simulink model "sampleModel1508"  (R2023a)
settings: Solver=VariableStepAuto  StartTime=0.0  StopTime=10.0  RelTol=1e-3
libraries: hdlsllib x4, simulink x3
settings Model: Creator=user1  LastModifiedBy=user1

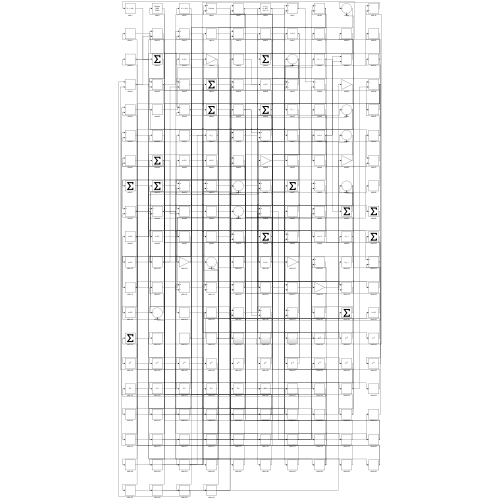
[thumbnail: Simulink's stored preview of the top-level diagram]
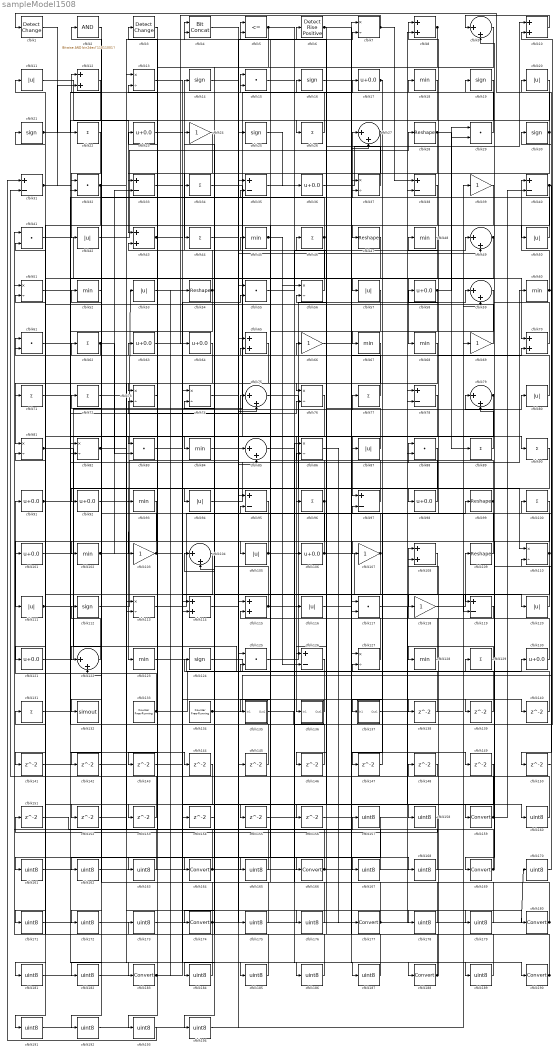
== system sampleModel1508 ==
  cfblk1 : simulink/Logic and Bit Operations/Detect Change  vinit=0  OutDataTypeStr=boolean
      settings: LibrarySourceBlock=|
      | hdlsllib/Logic and Bit
      | Operations/Detect
      | Change
  cfblk{8,10,12,43,65,70,108,114..115} (9 alike) : Sum
  cfblk{22,26,34,44,46,62,71..72,77,89..90,96,100,129,131} (15 alike) : Sum  Inputs=+
  cfblk{17,23,36,58,63..64,91..92,98,101,106,121,130} (13 alike) : Bias  Bias=0.0  SaturateOnIntegerOverflow=off
  cfblk{18,45,48,52,60,67..68,84,93,102,123,128} (12 alike) : MinMax
  cfblk{24,39,66,69,103,107,118} (7 alike) : Gain
  cfblk{9,27,49,59,75,79,85,104,122} (9 alike) : Sum  Inputs=|++
  cfblk{11,20,42,50,53,57,80,87,94,105,111,116,120} (13 alike) : Abs  SaturateOnIntegerOverflow=off
  cfblk{28,47,54,99,109} (5 alike) : Reshape
  cfblk{7,13,37,51,56,73..74,76,81..82,86,110,113,127} (14 alike) : Product  Inputs=*/  RndMeth=Zero  SaturateOnIntegerOverflow=on
  cfblk{14,16,19,21,25,30,112,124} (8 alike) : Signum
  cfblk{15,29,32,41,55,61,83,88,117,125} (10 alike) : DotProduct  OutDataTypeStr=Inherit: Inherit via internal rule
  cfblk{31,33,35,38,40,78,95,97,119,126} (10 alike) : Sum  Inputs=+-
  cfblk132 : ToWorkspace  VariableName=simout  SaveFormat=Timeseries  SampleTime=-1
  cfblk133 : hdlsllib/Sources/Counter Free-Running  NumBits=16  tsamp=-1
  cfblk134 : hdlsllib/Sources/Counter Free-Running  NumBits=16  tsamp=-1
  cfblk135 : Subsystem
      settings: LibrarySourceBlock=|
      | hdlsllib/Ports &
      | Subsystems/Subsystem
  cfblk136 : Subsystem
      settings: LibrarySourceBlock=|
      | hdlsllib/Ports &
      | Subsystems/Subsystem
  cfblk137 : Subsystem
      settings: LibrarySourceBlock=|
      | hdlsllib/Ports &
      | Subsystems/Subsystem
  cfblk{138..156} (19 alike) : Delay  SampleTime=1
  cfblk{157..158,160..163,165,167..168,170..173,175..176,178..179,181..182,184..187,189,191..194} (28 alike) : DataTypeConversion  OutDataTypeStr=uint8  SaturateOnIntegerOverflow=off  RndMeth=Floor
  cfblk{159,164,166,169,174,177,180,183,188,190} (10 alike) : DataTypeConversion  SaturateOnIntegerOverflow=off  RndMeth=Floor
  cfblk2 : simulink/Logic and Bit Operations/Bitwise Operator  logicop=AND  UseBitMask=on  BitMask=bin2dec('11011001')  BitMaskRealWorld=Stored Integer
      settings: LibrarySourceBlock=|
      | hdlsllib/Logic and Bit
      | Operations/Bitwise
      | Operator
  cfblk3 : simulink/Logic and Bit Operations/Detect Change  vinit=0  OutDataTypeStr=boolean
      settings: LibrarySourceBlock=|
      | hdlsllib/Logic and Bit
      | Operations/Detect
      | Change
  cfblk4 : hdlsllib/Logic and Bit Operations/Bit Concat  numInputs=2
  cfblk5 : RelationalOperator  Operator=<=  OutDataTypeStr=boolean  InputSameDT=off
  cfblk6 : hdlsllib/Logic and Bit Operations/Detect Rise Positive  vinit=0  OutDataTypeStr=boolean
  wires:
  cfblk66/1 -> cfblk188/1
  cfblk81/1 -> cfblk130/1, cfblk110/1
  cfblk25/1 -> cfblk36/1
  cfblk60/1 -> cfblk40/1, cfblk20/1
  cfblk49/1 -> cfblk68/1, cfblk137/1(In1)
  cfblk87/1 -> cfblk4/1
  cfblk54/1 -> cfblk14/1, cfblk82/2
  cfblk1/1 -> cfblk22/1
  cfblk124/1 -> cfblk129/1
  cfblk101/1 -> cfblk80/1
  cfblk70/1 -> cfblk16/1
  cfblk106/1 -> cfblk120/1, cfblk2/1
  cfblk134/1 -> cfblk30/1, cfblk37/2
  cfblk125/1 -> cfblk59/1
  cfblk137/1(Out1) -> cfblk69/1
  cfblk7/1 -> cfblk64/1, cfblk38/1
  cfblk50/1 -> cfblk27/1
  cfblk27/1 -> cfblk44/1, cfblk76/1
  cfblk17/1 -> cfblk47/1, cfblk67/1
  cfblk102/1 -> cfblk53/1, cfblk33/2
  cfblk136/1(Out1) -> cfblk24/1
  cfblk72/1 -> cfblk164/1
  cfblk133/1 -> cfblk91/1, cfblk75/2
  cfblk40/1 -> cfblk50/1, cfblk150/1, cfblk165/1, cfblk172/1
  cfblk37/1 -> cfblk6/1
  cfblk8/1 -> cfblk93/1, cfblk194/1
  cfblk64/1 -> cfblk81/1
  cfblk30/1 -> cfblk1/1, cfblk94/1
  cfblk45/1 -> cfblk56/1, cfblk126/2
  cfblk32/1 -> cfblk121/1, cfblk4/2
  cfblk43/1 -> cfblk90/1, cfblk143/1
  cfblk36/1 -> cfblk10/1
  cfblk24/1 -> cfblk83/1
  cfblk119/1 -> cfblk115/2
  cfblk118/1 -> cfblk109/1
  cfblk129/1 -> cfblk128/1
  cfblk80/1 -> cfblk48/1
  cfblk121/1 -> cfblk17/1
  cfblk77/1 -> cfblk61/1
  cfblk19/1 -> cfblk92/1
  cfblk103/1 -> cfblk62/1, cfblk55/2
  cfblk113/1 -> cfblk99/1
  cfblk6/1 -> cfblk26/1, cfblk160/1
  cfblk115/1 -> cfblk27/2, cfblk43/2
  cfblk105/1 -> cfblk102/1, cfblk38/2
  cfblk34/1 -> cfblk97/1
  cfblk56/1 -> cfblk34/1
  cfblk88/1 -> cfblk123/1
  cfblk28/1 -> cfblk107/1, cfblk89/1
  cfblk10/1 -> cfblk9/1
  cfblk41/1 -> cfblk70/1
  cfblk130/1 -> cfblk79/1
  cfblk22/1 -> cfblk42/1
  cfblk79/1 -> cfblk136/1(In1), cfblk106/1
  cfblk55/1 -> cfblk49/1
  cfblk9/1 -> cfblk96/1
  cfblk15/1 -> cfblk119/1
  cfblk42/1 -> cfblk28/1
  cfblk89/1 -> cfblk79/2
  cfblk128/1 -> cfblk108/1
  cfblk18/1 -> cfblk32/1
  cfblk51/1 -> cfblk183/1
  cfblk107/1 -> cfblk45/1, cfblk135/1(In1)
  cfblk13/1 -> cfblk166/1
  cfblk135/1(Out1) -> cfblk10/2
  cfblk21/1 -> cfblk15/1, cfblk57/1
  cfblk23/1 -> cfblk119/2
  cfblk112/1 -> cfblk25/1
  cfblk29/1 -> cfblk18/1
  cfblk82/1 -> cfblk187/1, cfblk189/1, cfblk192/1
  cfblk35/1 -> cfblk118/1
  cfblk20/1 -> cfblk116/1
  cfblk75/1 -> cfblk127/1
  cfblk92/1 -> cfblk77/1
  cfblk57/1 -> cfblk126/1
  cfblk94/1 -> cfblk60/1
  cfblk76/1 -> cfblk122/1
  cfblk111/1 -> cfblk21/1, cfblk88/1, cfblk41/2
  cfblk97/1 -> cfblk63/1
  cfblk61/1 -> cfblk98/1
  cfblk116/1 -> cfblk70/2
  cfblk98/1 -> cfblk5/1
  cfblk117/1 -> cfblk159/1
  cfblk47/1 -> cfblk105/1
  cfblk127/1 -> cfblk5/2
  cfblk12/1 -> cfblk32/2
  cfblk85/1 -> cfblk190/1
  cfblk123/1 -> cfblk127/2
  cfblk93/1 -> cfblk111/1
  cfblk73/1 -> cfblk103/1
  cfblk69/1 -> cfblk11/1
  cfblk120/1 -> cfblk19/1
  cfblk26/1 -> cfblk15/2
  cfblk5/1 -> cfblk33/1, cfblk139/1
  cfblk46/1 -> cfblk12/1, cfblk73/1
  cfblk48/1 -> cfblk71/1
  cfblk11/1 -> cfblk43/1
  cfblk86/1 -> cfblk177/1
  cfblk65/1 -> cfblk113/2
  cfblk99/1 -> cfblk8/1, cfblk156/1
  cfblk114/1 -> cfblk180/1
  cfblk58/1 -> cfblk29/1, cfblk29/2, cfblk155/1
  cfblk31/1 -> cfblk84/1, cfblk12/2
  cfblk110/1 -> cfblk58/1, cfblk184/1
  cfblk62/1 -> cfblk61/2, cfblk83/2
  cfblk44/1 -> cfblk49/2
  cfblk96/1 -> cfblk101/1, cfblk73/2
  cfblk2/1 -> cfblk132/1
  cfblk91/1 -> cfblk35/2, cfblk76/2
  cfblk109/1 -> cfblk3/1
  cfblk84/1 -> cfblk7/2
  cfblk100/1 -> cfblk169/1
  cfblk95/1 -> cfblk174/1
  cfblk126/1 -> cfblk125/2
  cfblk122/1 -> cfblk112/1
  cfblk83/1 -> cfblk138/1
  cfblk138/1 -> cfblk74/2
  cfblk139/1 -> cfblk56/2
  cfblk33/1 -> cfblk140/1
  cfblk140/1 -> cfblk7/1
  cfblk68/1 -> cfblk141/1
  cfblk90/1 -> cfblk142/1
  cfblk71/1 -> cfblk144/1
  cfblk4/1 -> cfblk145/1
  cfblk145/1 -> cfblk82/1
  cfblk59/1 -> cfblk146/1
  cfblk146/1 -> cfblk65/1
  cfblk108/1 -> cfblk147/1
  cfblk147/1 -> cfblk97/2
  cfblk148/1 -> cfblk31/2
  cfblk16/1 -> cfblk149/1
  cfblk150/1 -> cfblk110/2
  cfblk38/1 -> cfblk152/1
  cfblk152/1 -> cfblk113/1
  cfblk67/1 -> cfblk153/1
  cfblk153/1 -> cfblk81/2
  cfblk154/1 -> cfblk104/2
  cfblk155/1 -> cfblk8/2
  cfblk151/1 -> cfblk157/1
  cfblk53/1 -> cfblk158/1
  cfblk158/1 -> cfblk151/1
  cfblk159/1 -> cfblk46/1, cfblk40/2
  cfblk160/1 -> cfblk117/1
  cfblk157/1 -> cfblk161/1
  cfblk161/1 -> cfblk117/2
  cfblk52/1 -> cfblk162/1
  cfblk162/1 -> cfblk87/1
  cfblk3/1 -> cfblk163/1
  cfblk163/1 -> cfblk52/1
  cfblk164/1 -> cfblk59/2, cfblk41/1
  cfblk165/1 -> cfblk72/1
  cfblk166/1 -> cfblk75/1, cfblk104/1
  cfblk74/1 -> cfblk167/1
  cfblk167/1 -> cfblk13/1
  cfblk141/1 -> cfblk168/1
  cfblk168/1 -> cfblk13/2
  cfblk169/1 -> cfblk9/2, cfblk23/1
  cfblk170/1 -> cfblk100/1
  cfblk78/1 -> cfblk171/1
  cfblk171/1 -> cfblk115/1
  cfblk172/1 -> cfblk78/1
  cfblk173/1 -> cfblk78/2
  cfblk174/1 -> cfblk173/1, cfblk170/1, cfblk122/2
  cfblk14/1 -> cfblk175/1
  cfblk175/1 -> cfblk95/1
  cfblk142/1 -> cfblk176/1
  cfblk176/1 -> cfblk95/2
  cfblk177/1 -> cfblk88/2, cfblk74/1
  cfblk63/1 -> cfblk178/1
  cfblk178/1 -> cfblk86/1
  cfblk156/1 -> cfblk179/1
  cfblk179/1 -> cfblk86/2
  cfblk180/1 -> cfblk55/1, cfblk65/2
  cfblk104/1 -> cfblk181/1
  cfblk181/1 -> cfblk114/1
  cfblk144/1 -> cfblk182/1
  cfblk182/1 -> cfblk114/2
  cfblk183/1 -> cfblk154/1, cfblk54/1
  cfblk184/1 -> cfblk51/1
  cfblk143/1 -> cfblk185/1
  cfblk185/1 -> cfblk51/2
  cfblk131/1 -> cfblk186/1
  cfblk186/1 -> cfblk35/1
  cfblk187/1 -> cfblk131/1
  cfblk188/1 -> cfblk148/1, cfblk124/1, cfblk125/1
  cfblk189/1 -> cfblk66/1
  cfblk190/1 -> cfblk37/1, cfblk108/2
  cfblk149/1 -> cfblk191/1
  cfblk191/1 -> cfblk85/1
  cfblk192/1 -> cfblk85/2
  cfblk39/1 -> cfblk193/1
  cfblk193/1 -> cfblk31/1
  cfblk194/1 -> cfblk39/1

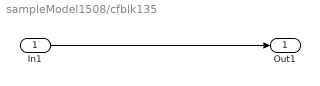
== system sampleModel1508/cfblk135 ==
  In1 : Inport
  Out1 : Outport
  wires:
  In1/1 -> Out1/1

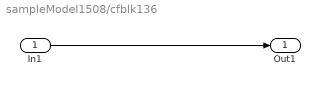
== system sampleModel1508/cfblk136 ==
  In1 : Inport
  Out1 : Outport
  wires:
  In1/1 -> Out1/1

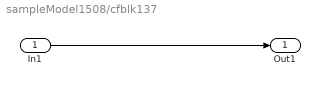
== system sampleModel1508/cfblk137 ==
  In1 : Inport
  Out1 : Outport
  wires:
  In1/1 -> Out1/1
